simulink model "sum5"  (R2020b)
settings: Solver=VariableStepAuto  StartTime=0.0  StopTime=10.0  RelTol=1e-3
undefined symbols (not defined in the file): C, R
settings Model: Creator=Shivani  LastModifiedBy=Shivani

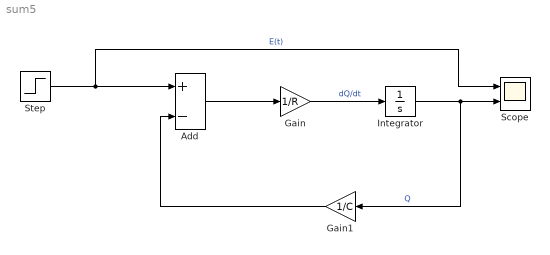
== system sum5 ==
  Add : Sum  Inputs=+-
  Gain : Gain  Gain=1/R
  Gain1 : Gain  Gain=1/C
  Integrator : Integrator  InitialCondition=5
  Scope : Scope  NumInputPorts=2
  Step : Step  Time=5  SampleTime=0
  wires:
  Step/1 -> Scope/1, Add/1  "E(t)"
  Add/1 -> Gain/1
  Gain/1 -> Integrator/1  "dQ/dt"
  Integrator/1 -> Gain1/1, Scope/2  "Q"
  Gain1/1 -> Add/2
